simulink model "model_inhibth_conditions_safety_module"  (R2024a)
settings: Solver=FixedStepAuto  StartTime=0.0  StopTime=10.0  RelTol=1e-3
libraries: simulink_extras x1
settings Model: Creator=Gabriel  LastModifiedBy=henri

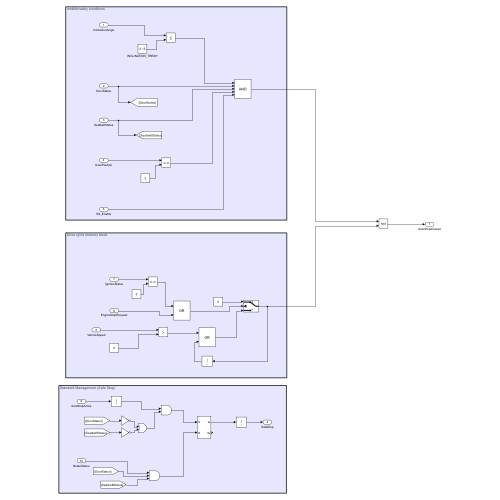
[thumbnail: Simulink's stored preview of the top-level diagram]
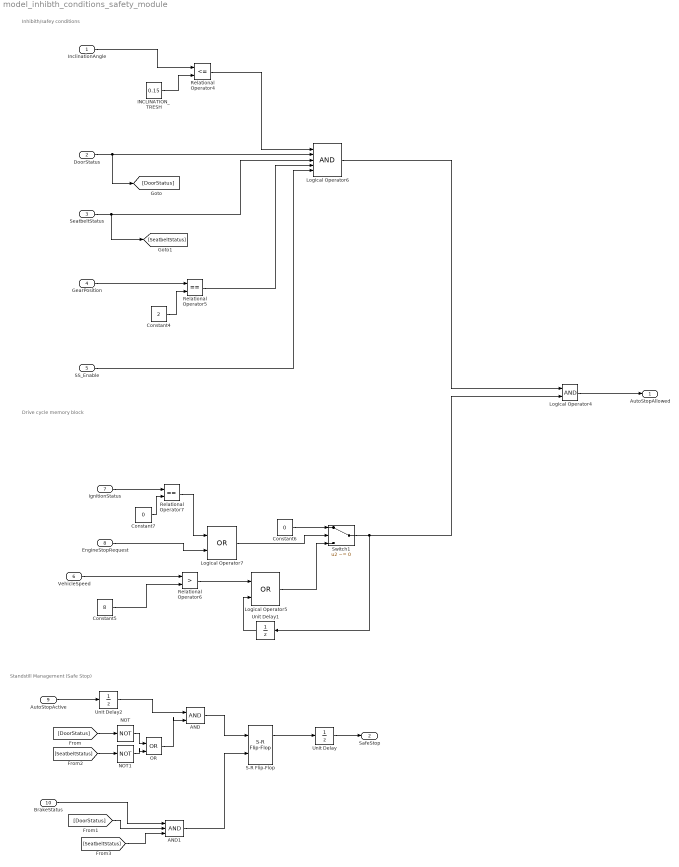
== system model_inhibth_conditions_safety_module ==
  note: Drive cycle memory block
  note: Inhibith/safey conditions
  note: Standstill Management (Safe Stop)
  InclinationAngle : Inport
  DoorStatus : Inport  Port=2
  SeatbeltStatus : Inport  Port=3
  GearPosition : Inport  Port=4
  SS_Enable : Inport  Port=5
  VehicleSpeed : Inport  Port=6
  IgnitionStatus : Inport  Port=7  OutDataTypeStr=boolean
  EngineStopRequest : Inport  Port=8
  AutoStopActive : Inport  Port=9
  BrakeStatus : Inport  Port=10
  AND : Logic  IconShape=distinctive  AllPortsSameDT=off  OutDataTypeStr=boolean
  AND1 : Logic  Inputs=3  IconShape=distinctive  AllPortsSameDT=off  OutDataTypeStr=boolean
  Constant4 : Constant  Value=2
  Constant5 : Constant  Value=8
  Constant6 : Constant  Value=0
  Constant7 : Constant  Value=0
  INCLINATION_TRESH : Constant  Value=0.15
  Logical Operator4 : Logic  AllPortsSameDT=off  OutDataTypeStr=boolean
  Logical Operator5 : Logic  Operator=OR  AllPortsSameDT=off  OutDataTypeStr=boolean
  Logical Operator6 : Logic  Inputs=5  AllPortsSameDT=off  OutDataTypeStr=boolean
  Logical Operator7 : Logic  Operator=OR  AllPortsSameDT=off  OutDataTypeStr=boolean
  NOT : Logic  Operator=NOT  IconShape=distinctive  AllPortsSameDT=off  OutDataTypeStr=boolean
  NOT1 : Logic  Operator=NOT  IconShape=distinctive  AllPortsSameDT=off  OutDataTypeStr=boolean
  OR : Logic  Operator=OR  IconShape=distinctive  AllPortsSameDT=off  OutDataTypeStr=boolean
  Relational Operator4 : RelationalOperator  Operator=<=  OutDataTypeStr=boolean  RndMeth=Simplest  InputSameDT=off
  Relational Operator5 : RelationalOperator  Operator===  OutDataTypeStr=boolean  RndMeth=Simplest  InputSameDT=off
  Relational Operator6 : RelationalOperator  Operator=>  OutDataTypeStr=boolean  RndMeth=Simplest  InputSameDT=off
  Relational Operator7 : RelationalOperator  Operator===  OutDataTypeStr=boolean  RndMeth=Simplest  InputSameDT=off
  S-R Flip-Flop : simulink_extras/Flip Flops/S-R Flip-Flop  initial_condition=0
  Switch1 : Switch  Criteria=u2 ~= 0  SaturateOnIntegerOverflow=off  InputSameDT=off
  Unit Delay : UnitDelay  SampleTime=0.1  HasFrameUpgradeWarning=on
  Unit Delay1 : UnitDelay  SampleTime=-1  HasFrameUpgradeWarning=on
  Unit Delay2 : UnitDelay  SampleTime=0.1  HasFrameUpgradeWarning=on
  AutoStopAllowed : Outport
  SafeStop : Outport  Port=2
  wires:
  SeatbeltStatus/1 -> [SeatbeltStatus], Logical Operator6/3
  INCLINATION_TRESH/1 -> Relational Operator4/2
  DoorStatus/1 -> [DoorStatus], Logical Operator6/2
  SS_Enable/1 -> Logical Operator6/5
  Relational Operator4/1 -> Logical Operator6/1
  InclinationAngle/1 -> Relational Operator4/1
  GearPosition/1 -> Relational Operator5/1
  Logical Operator6/1 -> Logical Operator4/1
  Relational Operator5/1 -> Logical Operator6/4
  Logical Operator4/1 -> AutoStopAllowed/1
  Switch1/1 -> Unit Delay1/1, Logical Operator4/2
  Logical Operator7/1 -> Switch1/2
  IgnitionStatus/1 -> Relational Operator7/1
  EngineStopRequest/1 -> Logical Operator7/2
  Unit Delay1/1 -> Logical Operator5/2
  Relational Operator7/1 -> Logical Operator7/1
  Constant7/1 -> Relational Operator7/2
  Relational Operator6/1 -> Logical Operator5/1
  VehicleSpeed/1 -> Relational Operator6/1
  Constant4/1 -> Relational Operator5/2
  Constant5/1 -> Relational Operator6/2
  Logical Operator5/1 -> Switch1/3
  Constant6/1 -> Switch1/1
  AutoStopActive/1 -> Unit Delay2/1
  [DoorStatus] -> NOT/1
  AND/1 -> S-R Flip-Flop/1
  BrakeStatus/1 -> AND1/1
  AND1/1 -> S-R Flip-Flop/2
  S-R Flip-Flop/1 -> Unit Delay/1
  Unit Delay/1 -> SafeStop/1
  [DoorStatus] -> AND1/2
  [SeatbeltStatus] -> NOT1/1
  NOT/1 -> OR/1
  NOT1/1 -> OR/2
  OR/1 -> AND/2
  Unit Delay2/1 -> AND/1
  [SeatbeltStatus] -> AND1/3
